simulink model "admittance_controller_euler"  (R2021b)
settings: Solver=VariableStepAuto  StartTime=0.0  StopTime=10.0  RelTol=1e-3
undefined symbols (not defined in the file): ddphi_d, dphi_d, mu, phi_d
settings Model: Creator=Martin  LastModifiedBy=Martin

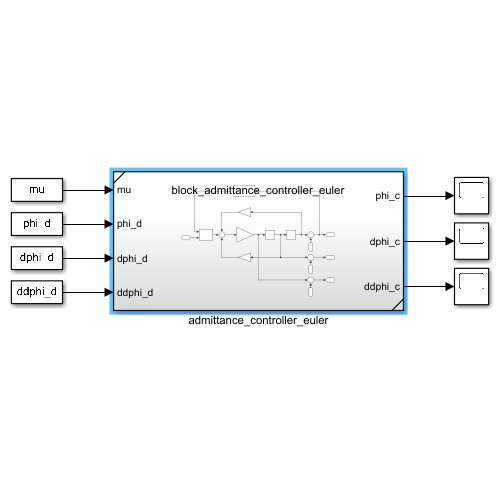
[thumbnail: Simulink's stored preview of the top-level diagram]
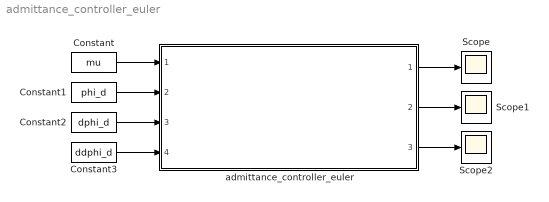
== system admittance_controller_euler ==
  Constant : Constant  Value=mu  VectorParams1D=off
  Constant1 : Constant  Value=phi_d  VectorParams1D=off
  Constant2 : Constant  Value=dphi_d  VectorParams1D=off
  Constant3 : Constant  Value=ddphi_d  VectorParams1D=off
  Scope : Scope
  Scope1 : Scope
  Scope2 : Scope
  admittance_controller_euler : Subsystem  ReferencedSubsystem=block_admittance_controller_euler
  wires:
  Constant/1 -> admittance_controller_euler/1
  Constant1/1 -> admittance_controller_euler/2
  Constant2/1 -> admittance_controller_euler/3
  Constant3/1 -> admittance_controller_euler/4
  admittance_controller_euler/1 -> Scope/1
  admittance_controller_euler/2 -> Scope1/1
  admittance_controller_euler/3 -> Scope2/1
